simulink model "sliding_mode"  (R2025b)
settings: Solver=VariableStepAuto  StartTime=0.0  StopTime=200  RelTol=1e-3
libraries: simulink x3, matrix_library x1
settings Model: SimulationMode=rapid-accelerator  Creator=srivatsan  LastModifiedBy=srivatsan

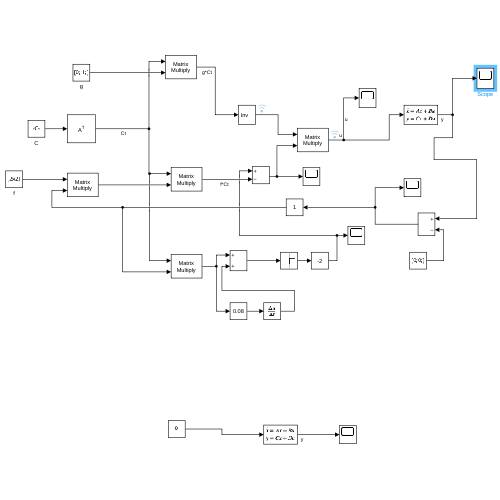
[thumbnail: Simulink's stored preview of the top-level diagram]
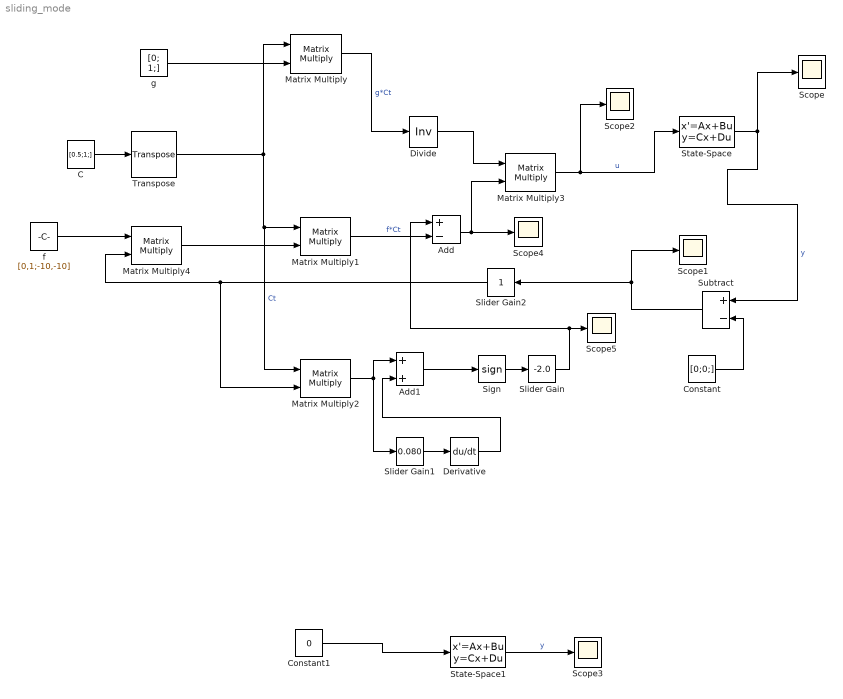
== system sliding_mode ==
  Add : Sum  Inputs=+-
  Add1 : Sum
  C : Constant  Value=[0.5;1;]
  Constant : Constant  Value=[0;0;]  VectorParams1D=off
  Constant1 : Constant  Value=0
  Derivative : Derivative
  Divide : Product  Inputs=/  Multiplication=Matrix(*)
  Matrix Multiply{,1..4} (5 alike) : Product  Multiplication=Matrix(*)
  Scope{,1..5} (6 alike) : Scope
      Scope settings: ActiveDisplayYMinimum=-3.235311047047833  ActiveDisplayYMaximum=7.6043260758039981
      Scope1 settings: ActiveDisplayYMinimum=-1112.590087174824  ActiveDisplayYMaximum=128.25322416692461
      Scope2 settings: ActiveDisplayYMinimum=74.159125396484782  ActiveDisplayYMaximum=78.348664860808  DataLoggingVariableName=ScopeData2
      Scope3 settings: ActiveDisplayYMinimum=-7.1016769488332123  ActiveDisplayYMaximum=3.4136978035141685  DataLoggingVariableName=ScopeData3
      Scope4 settings: ActiveDisplayYMinimum=-6382.9421893122317  ActiveDisplayYMaximum=-6260.811247975751  DataLoggingVariableName=ScopeData4
      Scope5 settings: ActiveDisplayYMinimum=-0.88939595921260117  ActiveDisplayYMaximum=-0.73873024916599506  DataLoggingVariableName=ScopeData5
  Sign : Signum  ZeroCross=off
  Slider Gain : simulink/Math Operations/Slider Gain  gain=-2.0  low=-2  high=2
  Slider Gain1 : simulink/Math Operations/Slider Gain  gain=0.080  low=-2  high=2
  Slider Gain2 : simulink/Math Operations/Slider Gain  gain=1  low=-2  high=2
  State-Space : StateSpace  A=[0,1;-10,-10]  B=[0;1;]  C=eye(2)  D=zeros(2,1)  InitialCondition=[5;3;]
  State-Space1 : StateSpace  A=[0,1;-10,-10]  B=[0;1;]  C=eye(2)  D=zeros(2,1)  InitialCondition=[5;3;]
  Subtract : Sum  Inputs=+-
  Transpose : matrix_library/Transpose
  f : Constant  Value=[0,1;-10,-10]
  g : Constant  Value=[0; 1;]  VectorParams1D=off
  wires:
  C/1 -> Transpose/1
  Transpose/1 -> Matrix Multiply/1, Matrix Multiply2/1, Matrix Multiply1/1  "Ct"
  g/1 -> Matrix Multiply/2
  State-Space/1 -> Subtract/1, Scope/1  "y"
  Sign/1 -> Slider Gain/1
  Matrix Multiply1/1 -> Add/2  "f*Ct"
  Divide/1 -> Matrix Multiply3/1
  Add/1 -> Matrix Multiply3/2, Scope4/1
  Matrix Multiply/1 -> Divide/1  "g*Ct"
  f/1 -> Matrix Multiply4/1
  Matrix Multiply4/1 -> Matrix Multiply1/2
  Subtract/1 -> Scope1/1, Slider Gain2/1
  Slider Gain2/1 -> Matrix Multiply2/2, Matrix Multiply4/2
  Matrix Multiply2/1 -> Slider Gain1/1, Add1/1
  Slider Gain1/1 -> Derivative/1
  Derivative/1 -> Add1/2
  Add1/1 -> Sign/1
  Matrix Multiply3/1 -> Scope2/1, State-Space/1  "u"
  Constant/1 -> Subtract/2
  Constant1/1 -> State-Space1/1
  State-Space1/1 -> Scope3/1  "y"
  Slider Gain/1 -> Add/1, Scope5/1
